simulink model "Double_Pendulum_Project"  (R2021a)
settings: Solver=ode4  StartTime=0.0  StopTime=50  FixedStep=0.001  RelTol=1e-3
settings Model: Creator=YW  LastModifiedBy=YW

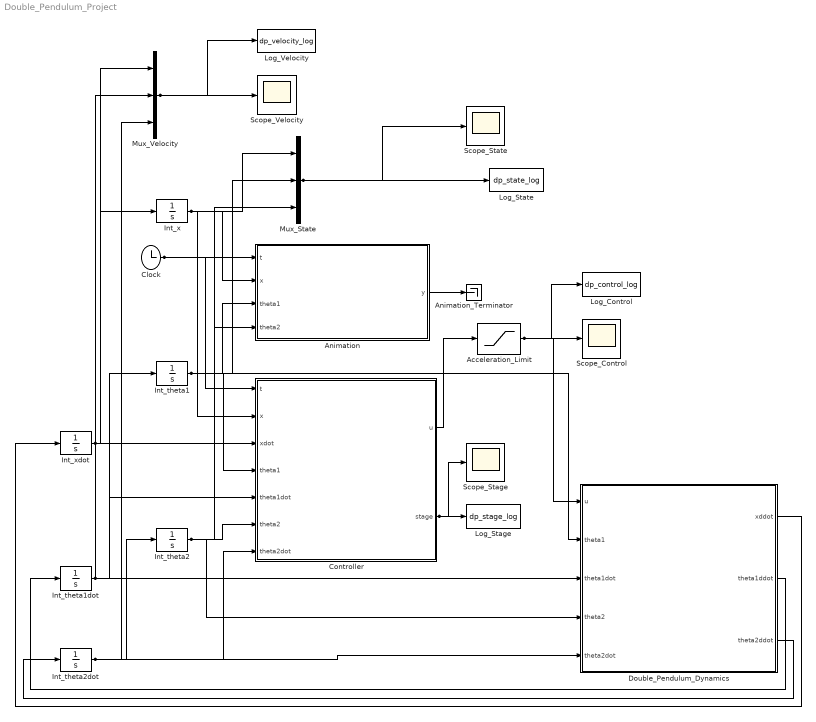
== system Double_Pendulum_Project ==
  Acceleration_Limit : Saturate  UpperLimit=30  LowerLimit=-30
  Animation : MATLAB Function  TreatAsAtomicUnit=on
  Animation_Terminator : Terminator
  Clock : Clock
  Controller : MATLAB Function  TreatAsAtomicUnit=on  SystemSampleTime=0.001
  Double_Pendulum_Dynamics : MATLAB Function  TreatAsAtomicUnit=on
  Int_theta1 : Integrator  InitialCondition=3.0616
  Int_theta1dot : Integrator
  Int_theta2 : Integrator  InitialCondition=-3.0816
  Int_theta2dot : Integrator
  Int_x : Integrator
  Int_xdot : Integrator
  Log_Control : ToWorkspace  VariableName=dp_control_log  SaveFormat=Structure With Time  SampleTime=-1
  Log_Stage : ToWorkspace  VariableName=dp_stage_log  SaveFormat=Structure With Time  SampleTime=-1
  Log_State : ToWorkspace  VariableName=dp_state_log  SaveFormat=Structure With Time  SampleTime=-1
  Log_Velocity : ToWorkspace  VariableName=dp_velocity_log  SaveFormat=Structure With Time  SampleTime=-1
  Mux_State : Mux  Inputs=3
  Mux_Velocity : Mux  Inputs=3
  Scope_Control : Scope
  Scope_Stage : Scope
  Scope_State : Scope
  Scope_Velocity : Scope
  wires:
  Animation/1(y) -> Animation_Terminator/1
  Double_Pendulum_Dynamics/3(theta2ddot) -> Int_theta2dot/1
  Acceleration_Limit/1 -> Double_Pendulum_Dynamics/1(u), Scope_Control/1, Log_Control/1
  Int_theta2/1 -> Double_Pendulum_Dynamics/4(theta2), Controller/6(theta2), Mux_State/3, Animation/4(theta2)
  Mux_State/1 -> Scope_State/1, Log_State/1
  Int_theta2dot/1 -> Int_theta2/1, Double_Pendulum_Dynamics/5(theta2dot), Controller/7(theta2dot), Mux_Velocity/3
  Clock/1 -> Controller/1(t), Animation/1(t)
  Mux_Velocity/1 -> Scope_Velocity/1, Log_Velocity/1
  Double_Pendulum_Dynamics/2(theta1ddot) -> Int_theta1dot/1
  Double_Pendulum_Dynamics/1(xddot) -> Int_xdot/1
  Controller/1(u) -> Acceleration_Limit/1
  Controller/2(stage) -> Scope_Stage/1, Log_Stage/1
  Int_theta1/1 -> Double_Pendulum_Dynamics/2(theta1), Controller/4(theta1), Mux_State/2, Animation/3(theta1)
  Int_x/1 -> Controller/2(x), Mux_State/1, Animation/2(x)
  Int_xdot/1 -> Int_x/1, Controller/3(xdot), Mux_Velocity/1
  Int_theta1dot/1 -> Int_theta1/1, Double_Pendulum_Dynamics/3(theta1dot), Controller/5(theta1dot), Mux_Velocity/2

== matlab function Double_Pendulum_Project/Double_Pendulum_Dynamics ==
  data: u input; xddot output; theta1 input; theta1dot input; theta2 input; theta2dot input; theta1ddot output; theta2ddot output
function [xddot,theta1ddot,theta2ddot] = fcn(u,theta1,theta1dot,theta2,theta2dot)
[xddot,theta1ddot,theta2ddot] = dp_dynamics(u,theta1,theta1dot,theta2,theta2dot);
end

== matlab function Double_Pendulum_Project/Controller ==
  data: t input; u output; x input; xdot input; theta1 input; theta1dot input; theta2 input; theta2dot input; stage output
function [u,stage] = fcn(t,x,xdot,theta1,theta1dot,theta2,theta2dot)
[u,stage] = dp_controller(t,x,xdot,theta1,theta1dot,theta2,theta2dot);
end

== matlab function Double_Pendulum_Project/Animation ==
  data: t input; y output; x input; theta1 input; theta2 input
function y = fcn(t,x,theta1,theta2)
y = 0*t + 0*x + 0*theta1 + 0*theta2;
end
